simulink model "TTS2_EXT"  (R2025b)
settings: Solver=FixedStepAuto  StartTime=0.0  StopTime=inf  FixedStep=0.01  RelTol=1e-3
model workspace (MAT data in the model file):
  amp_f1 = -100
  amp_f10 = 0.5
  amp_f11 = -0.1
  amp_f12 = 1
  amp_f13 = 0.5
  amp_f14 = -20
  amp_f15 = 0.5
  amp_f16 = 0.5
  amp_f17 = 20
  amp_f18 = -30
  amp_f19 = 0.1
  amp_f2 = -20
  amp_f20 = -20
  amp_f21 = 20
  amp_f3 = -30
  amp_f4 = -30
  amp_f5 = -10
  amp_f51 = -10
  amp_f52 = -30
  amp_f53 = -30
  amp_f54 = 20
  amp_f55 = -100
  amp_f6 = -30
  amp_f7 = -30
  amp_f8 = -30
  amp_f9 = 1
  from_f1 = 570
  from_f10 = 5970
  from_f11 = 6570
  from_f12 = 7170
  from_f13 = 7770
  from_f14 = 8370
  from_f15 = 8970
  from_f16 = 9570
  from_f17 = 10170
  from_f18 = 10770
  from_f19 = 11370
  from_f2 = 1170
  from_f20 = 11970
  from_f21 = 12570
  from_f3 = 1770
  from_f4 = 2370
  from_f5 = 2970
  from_f51 = 13170
  from_f52 = 13770
  from_f53 = 14370
  from_f54 = 14970
  from_f55 = 15570
  from_f6 = 3570
  from_f7 = 4170
  from_f8 = 4770
  from_f9 = 5370
libraries: lab310_library x26, neural x15, simulink x4, opclib x3, fuzblock x1
(part 3 of 3)

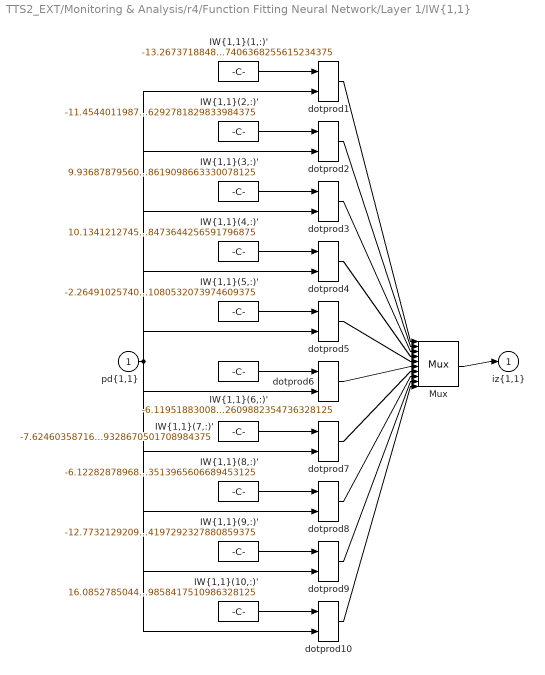
== system TTS2_EXT/Monitoring & Analysis/r4/Function Fitting Neural Network/Layer 1/IW{1,1} ==
  "pd{1,1}" : Inport  PortDimensions=1
      mask Display: e = 0.06;c1 = [120 230 180]/255;c2 = ([120 230 180]+0)/(256+128);c3 = ([120 230 180]+128)/(256+128);patch([0 1 1 0],[0 0 1 1],c1);patch([0 1 1 1-e 1-e 0+e],[0 0 1 1-e 0+e 0+e],c2);patch([0 0 1 1-e 0+e 0+e],[0 1 1 1-e 1-e 0+e],c3);plot([0 1 1 0 0],[0 0 1 1 0]);
  "IW{1,1}(1,:)'" : Constant  Value=-13.267371884858700781251172884367406368255615234375
      mask Display: e = 0.06;c1 = [120 150 230]/255;c2 = ([120 150 230]+0)/383;c3 = ([120 150 230]+128)/383;patch([0 1 1 0],[0 0 1 1],c1);patch([0 1 1 1-e 1-e 0+e],[0 0 1 1-e 0+e 0+e],c2);patch([0 0 1 1-e 0+e 0+e],[0 1 1 1-e 1-e 0+e],c3);plot([0 1 1 0 0],[0 0 1 1 0]);disp('Weights');
  "IW{1,1}(10,:)'" : Constant  Value=16.085278504446240077641050447709858417510986328125
      mask Display: e = 0.06;c1 = [120 150 230]/255;c2 = ([120 150 230]+0)/383;c3 = ([120 150 230]+128)/383;patch([0 1 1 0],[0 0 1 1],c1);patch([0 1 1 1-e 1-e 0+e],[0 0 1 1-e 0+e 0+e],c2);patch([0 0 1 1-e 0+e 0+e],[0 1 1 1-e 1-e 0+e],c3);plot([0 1 1 0 0],[0 0 1 1 0]);disp('Weights');
  "IW{1,1}(2,:)'" : Constant  Value=-11.4544011987529952278919154196046292781829833984375
      mask Display: e = 0.06;c1 = [120 150 230]/255;c2 = ([120 150 230]+0)/383;c3 = ([120 150 230]+128)/383;patch([0 1 1 0],[0 0 1 1],c1);patch([0 1 1 1-e 1-e 0+e],[0 0 1 1-e 0+e 0+e],c2);patch([0 0 1 1-e 0+e 0+e],[0 1 1 1-e 1-e 0+e],c3);plot([0 1 1 0 0],[0 0 1 1 0]);disp('Weights');
  "IW{1,1}(3,:)'" : Constant  Value=9.936878795604048519862772081978619098663330078125
      mask Display: e = 0.06;c1 = [120 150 230]/255;c2 = ([120 150 230]+0)/383;c3 = ([120 150 230]+128)/383;patch([0 1 1 0],[0 0 1 1],c1);patch([0 1 1 1-e 1-e 0+e],[0 0 1 1-e 0+e 0+e],c2);patch([0 0 1 1-e 0+e 0+e],[0 1 1 1-e 1-e 0+e],c3);plot([0 1 1 0 0],[0 0 1 1 0]);disp('Weights');
  "IW{1,1}(4,:)'" : Constant  Value=10.1341212745394653182984257000498473644256591796875
      mask Display: e = 0.06;c1 = [120 150 230]/255;c2 = ([120 150 230]+0)/383;c3 = ([120 150 230]+128)/383;patch([0 1 1 0],[0 0 1 1],c1);patch([0 1 1 1-e 1-e 0+e],[0 0 1 1-e 0+e 0+e],c2);patch([0 0 1 1-e 0+e 0+e],[0 1 1 1-e 1-e 0+e],c3);plot([0 1 1 0 0],[0 0 1 1 0]);disp('Weights');
  "IW{1,1}(5,:)'" : Constant  Value=-2.26491025740641926944363149232231080532073974609375
      mask Display: e = 0.06;c1 = [120 150 230]/255;c2 = ([120 150 230]+0)/383;c3 = ([120 150 230]+128)/383;patch([0 1 1 0],[0 0 1 1],c1);patch([0 1 1 1-e 1-e 0+e],[0 0 1 1-e 0+e 0+e],c2);patch([0 0 1 1-e 0+e 0+e],[0 1 1 1-e 1-e 0+e],c3);plot([0 1 1 0 0],[0 0 1 1 0]);disp('Weights');
  "IW{1,1}(6,:)'" : Constant  Value=-6.1195188300888077037598122842609882354736328125
      mask Display: e = 0.06;c1 = [120 150 230]/255;c2 = ([120 150 230]+0)/383;c3 = ([120 150 230]+128)/383;patch([0 1 1 0],[0 0 1 1],c1);patch([0 1 1 1-e 1-e 0+e],[0 0 1 1-e 0+e 0+e],c2);patch([0 0 1 1-e 0+e 0+e],[0 1 1 1-e 1-e 0+e],c3);plot([0 1 1 0 0],[0 0 1 1 0]);disp('Weights');
  "IW{1,1}(7,:)'" : Constant  Value=-7.62460358716090436104195759980939328670501708984375
      mask Display: e = 0.06;c1 = [120 150 230]/255;c2 = ([120 150 230]+0)/383;c3 = ([120 150 230]+128)/383;patch([0 1 1 0],[0 0 1 1],c1);patch([0 1 1 1-e 1-e 0+e],[0 0 1 1-e 0+e 0+e],c2);patch([0 0 1 1-e 0+e 0+e],[0 1 1 1-e 1-e 0+e],c3);plot([0 1 1 0 0],[0 0 1 1 0]);disp('Weights');
  "IW{1,1}(8,:)'" : Constant  Value=-6.122828789688373518629305181093513965606689453125
      mask Display: e = 0.06;c1 = [120 150 230]/255;c2 = ([120 150 230]+0)/383;c3 = ([120 150 230]+128)/383;patch([0 1 1 0],[0 0 1 1],c1);patch([0 1 1 1-e 1-e 0+e],[0 0 1 1-e 0+e 0+e],c2);patch([0 0 1 1-e 0+e 0+e],[0 1 1 1-e 1-e 0+e],c3);plot([0 1 1 0 0],[0 0 1 1 0]);disp('Weights');
  "IW{1,1}(9,:)'" : Constant  Value=-12.7732129209851503759409752092324197292327880859375
      mask Display: e = 0.06;c1 = [120 150 230]/255;c2 = ([120 150 230]+0)/383;c3 = ([120 150 230]+128)/383;patch([0 1 1 0],[0 0 1 1],c1);patch([0 1 1 1-e 1-e 0+e],[0 0 1 1-e 0+e 0+e],c2);patch([0 0 1 1-e 0+e 0+e],[0 1 1 1-e 1-e 0+e],c3);plot([0 1 1 0 0],[0 0 1 1 0]);disp('Weights');
  Mux : Mux  Inputs=10
      mask Display: e = 0.06;c1 = [120 150 230]/255;c2 = ([120 150 230]+0)/383;c3 = ([120 150 230]+128)/383;patch([0 1 1 0],[0 0 1 1],c1);patch([0 1 1 1-e 1-e 0+e],[0 0 1 1-e 0+e 0+e],c2);patch([0 0 1 1-e 0+e 0+e],[0 1 1 1-e 1-e 0+e],c3);plot([0 1 1 0 0],[0 0 1 1 0]);disp('Mux');
  dotprod{1..10} (10 alike) : neural/Weight Functions/dotprod
  "iz{1,1}" : Outport
      mask Display: e = 0.06;c1 = [120 230 180]/255;c2 = ([120 230 180]+0)/(256+128);c3 = ([120 230 180]+128)/(256+128);patch([0 1 1 0],[0 0 1 1],c1);patch([0 1 1 1-e 1-e 0+e],[0 0 1 1-e 0+e 0+e],c2);patch([0 0 1 1-e 0+e 0+e],[0 1 1 1-e 1-e 0+e],c3);plot([0 1 1 0 0],[0 0 1 1 0]);
  wires:
  "IW{1,1}(1,:)'"/1 -> dotprod1/1
  "pd{1,1}"/1 -> dotprod1/2, dotprod2/2, dotprod3/2, dotprod4/2, dotprod5/2, dotprod6/2, dotprod7/2, dotprod8/2, dotprod9/2, dotprod10/2
  dotprod1/1 -> Mux/1
  "IW{1,1}(2,:)'"/1 -> dotprod2/1
  dotprod2/1 -> Mux/2
  "IW{1,1}(3,:)'"/1 -> dotprod3/1
  dotprod3/1 -> Mux/3
  "IW{1,1}(4,:)'"/1 -> dotprod4/1
  dotprod4/1 -> Mux/4
  "IW{1,1}(5,:)'"/1 -> dotprod5/1
  dotprod5/1 -> Mux/5
  "IW{1,1}(6,:)'"/1 -> dotprod6/1
  dotprod6/1 -> Mux/6
  "IW{1,1}(7,:)'"/1 -> dotprod7/1
  dotprod7/1 -> Mux/7
  "IW{1,1}(8,:)'"/1 -> dotprod8/1
  dotprod8/1 -> Mux/8
  "IW{1,1}(9,:)'"/1 -> dotprod9/1
  dotprod9/1 -> Mux/9
  "IW{1,1}(10,:)'"/1 -> dotprod10/1
  dotprod10/1 -> Mux/10
  Mux/1 -> "iz{1,1}"/1

== system TTS2_EXT/Monitoring & Analysis/r4/Function Fitting Neural Network/Layer 2/Delays 1 ==
  "p{2}" : Inport  PortDimensions=10
      mask Display: e = 0.06;c1 = [120 230 180]/255;c2 = ([120 230 180]+0)/(256+128);c3 = ([120 230 180]+128)/(256+128);patch([0 1 1 0],[0 0 1 1],c1);patch([0 1 1 1-e 1-e 0+e],[0 0 1 1-e 0+e 0+e],c2);patch([0 0 1 1-e 0+e 0+e],[0 1 1 1-e 1-e 0+e],c3);plot([0 1 1 0 0],[0 0 1 1 0]);
  mux : Mux  Inputs=1
      mask Display: e = 0.06;c1 = [120 150 230]/255;c2 = ([120 150 230]+0)/383;c3 = ([120 150 230]+128)/383;patch([0 1 1 0],[0 0 1 1],c1);patch([0 1 1 1-e 1-e 0+e],[0 0 1 1-e 0+e 0+e],c2);patch([0 0 1 1-e 0+e 0+e],[0 1 1 1-e 1-e 0+e],c3);plot([0 1 1 0 0],[0 0 1 1 0]);disp('Mux')
  "pd{2,1}" : Outport
      mask Display: e = 0.06;c1 = [120 230 180]/255;c2 = ([120 230 180]+0)/(256+128);c3 = ([120 230 180]+128)/(256+128);patch([0 1 1 0],[0 0 1 1],c1);patch([0 1 1 1-e 1-e 0+e],[0 0 1 1-e 0+e 0+e],c2);patch([0 0 1 1-e 0+e 0+e],[0 1 1 1-e 1-e 0+e],c3);plot([0 1 1 0 0],[0 0 1 1 0]);
  wires:
  "p{2}"/1 -> mux/1
  mux/1 -> "pd{2,1}"/1

== system TTS2_EXT/Monitoring & Analysis/r4/Function Fitting Neural Network/Layer 2/LW{2,1} ==
  "ad{2,1}" : Inport  PortDimensions=10
      mask Display: e = 0.06;c1 = [120 230 180]/255;c2 = ([120 230 180]+0)/(256+128);c3 = ([120 230 180]+128)/(256+128);patch([0 1 1 0],[0 0 1 1],c1);patch([0 1 1 1-e 1-e 0+e],[0 0 1 1-e 0+e 0+e],c2);patch([0 0 1 1-e 0+e 0+e],[0 1 1 1-e 1-e 0+e],c3);plot([0 1 1 0 0],[0 0 1 1 0]);
  "IW{2,1}(1,:)'" : Constant  Value=[-0.0273434432413987814347589022645479417406022548675537109375;-0.04215844327802921454040330218049348331987857818603515625;0.0296321635772760529070612989244182244874536991119384765625;0.019112043841627852913678253798934747464954853057861328125;-0.282504725481045382284861489097238518297672271728515625;-0.0481063819827808047957518056136905215680599212646484375;-0.06977041381876440684361995181461679749190807342529296875;-0.179432033501076226844617167444084770977497100830078125;-0.10706544318229176127044155464318464510142803192138671875;1.657272038694669991087948801578022539615631103515625]
      mask Display: e = 0.06;c1 = [120 150 230]/255;c2 = ([120 150 230]+0)/383;c3 = ([120 150 230]+128)/383;patch([0 1 1 0],[0 0 1 1],c1);patch([0 1 1 1-e 1-e 0+e],[0 0 1 1-e 0+e 0+e],c2);patch([0 0 1 1-e 0+e 0+e],[0 1 1 1-e 1-e 0+e],c3);plot([0 1 1 0 0],[0 0 1 1 0]);disp('weights');
  Mux : Mux  Inputs=1
      mask Display: e = 0.06;c1 = [120 150 230]/255;c2 = ([120 150 230]+0)/383;c3 = ([120 150 230]+128)/383;patch([0 1 1 0],[0 0 1 1],c1);patch([0 1 1 1-e 1-e 0+e],[0 0 1 1-e 0+e 0+e],c2);patch([0 0 1 1-e 0+e 0+e],[0 1 1 1-e 1-e 0+e],c3);plot([0 1 1 0 0],[0 0 1 1 0]);disp('Mux');
  dotprod1 : neural/Weight Functions/dotprod
  "lz{2,1}" : Outport
      mask Display: e = 0.06;c1 = [120 230 180]/255;c2 = ([120 230 180]+0)/(256+128);c3 = ([120 230 180]+128)/(256+128);patch([0 1 1 0],[0 0 1 1],c1);patch([0 1 1 1-e 1-e 0+e],[0 0 1 1-e 0+e 0+e],c2);patch([0 0 1 1-e 0+e 0+e],[0 1 1 1-e 1-e 0+e],c3);plot([0 1 1 0 0],[0 0 1 1 0]);
  wires:
  "IW{2,1}(1,:)'"/1 -> dotprod1/1
  "ad{2,1}"/1 -> dotprod1/2
  dotprod1/1 -> Mux/1
  Mux/1 -> "lz{2,1}"/1

== system TTS2_EXT/TTS2/Disturbance: Pump+pipe+control valve/VB/Valve/liniowa ==
  CV : Inport
  dP : Inport  Port=2
  param : Inport  Port=3
  Bus Selector : BusSelector  OutputSignals=signal4,signal2,signal1,signal3
  Fcn : Fcn  Expr=u(2)*(u(1)-1)
  Fcn1 : Fcn  Expr=sqrt(u(1)/u(2))/10
  Math Function : Math  SignedPower=on
  Mux : Mux  Inputs=2
  Mux1 : Mux  Inputs=2
  Product : Product  Inputs=*/***
  F : Outport  VectorParamsAs1DForOutWhenUnconnected=off
  wires:
  param/1 -> Bus Selector/1
  Fcn/1 -> Math Function/1
  Math Function/1 -> Product/1
  Product/1 -> F/1
  Mux/1 -> Fcn/1
  Mux1/1 -> Fcn1/1
  dP/1 -> Mux1/1
  Bus Selector/2 -> Mux/2  "<signal2>"
  Bus Selector/3 -> Product/3  "<signal1>"
  Fcn1/1 -> Product/5
  Bus Selector/4 -> Mux1/2  "<signal3>"
  Bus Selector/1 -> Product/2, Mux/1  "<signal4>"
  CV/1 -> Product/4

== system TTS2_EXT/TTS2/Disturbance: Pump+pipe+control valve/VB/Valve/stałoproc. ==
  CV : Inport
  dP : Inport  Port=2
  param : Inport  Port=3
  Bus Selector : BusSelector  OutputSignals=signal2,signal1,signal3
  Fcn : Fcn  Expr=u(2)*(u(1)-1)
  Fcn1 : Fcn  Expr=sqrt(u(1)/u(2))/10
  Math Function : Math  SignedPower=on
  Mux : Mux  Inputs=2
  Mux1 : Mux  Inputs=2
  Product : Product  Inputs=3
  F : Outport  VectorParamsAs1DForOutWhenUnconnected=off
  wires:
  param/1 -> Bus Selector/1
  Fcn/1 -> Math Function/1
  Math Function/1 -> Product/1
  Product/1 -> F/1
  CV/1 -> Mux/1
  Mux/1 -> Fcn/1
  Mux1/1 -> Fcn1/1
  dP/1 -> Mux1/1
  Bus Selector/1 -> Mux/2  "<signal2>"
  Bus Selector/2 -> Product/2  "<signal1>"
  Fcn1/1 -> Product/3
  Bus Selector/3 -> Mux1/2  "<signal3>"

== system TTS2_EXT/TTS2/Pump+pipe+control valve/V1/Valve/liniowa ==
  CV : Inport
  dP : Inport  Port=2
  param : Inport  Port=3
  Bus Selector : BusSelector  OutputSignals=signal4,signal2,signal1,signal3
  Fcn : Fcn  Expr=u(2)*(u(1)-1)
  Fcn1 : Fcn  Expr=sqrt(u(1)/u(2))/10
  Math Function : Math  SignedPower=on
  Mux : Mux  Inputs=2
  Mux1 : Mux  Inputs=2
  Product : Product  Inputs=*/***
  F : Outport  VectorParamsAs1DForOutWhenUnconnected=off
  wires:
  param/1 -> Bus Selector/1
  Fcn/1 -> Math Function/1
  Math Function/1 -> Product/1
  Product/1 -> F/1
  Mux/1 -> Fcn/1
  Mux1/1 -> Fcn1/1
  dP/1 -> Mux1/1
  Bus Selector/2 -> Mux/2  "<signal2>"
  Bus Selector/3 -> Product/3  "<signal1>"
  Fcn1/1 -> Product/5
  Bus Selector/4 -> Mux1/2  "<signal3>"
  Bus Selector/1 -> Product/2, Mux/1  "<signal4>"
  CV/1 -> Product/4

== system TTS2_EXT/TTS2/Pump+pipe+control valve/V1/Valve/stałoproc. ==
  CV : Inport
  dP : Inport  Port=2
  param : Inport  Port=3
  Bus Selector : BusSelector  OutputSignals=signal2,signal1,signal3
  Fcn : Fcn  Expr=u(2)*(u(1)-1)
  Fcn1 : Fcn  Expr=sqrt(u(1)/u(2))/10
  Math Function : Math  SignedPower=on
  Mux : Mux  Inputs=2
  Mux1 : Mux  Inputs=2
  Product : Product  Inputs=3
  F : Outport  VectorParamsAs1DForOutWhenUnconnected=off
  wires:
  param/1 -> Bus Selector/1
  Fcn/1 -> Math Function/1
  Math Function/1 -> Product/1
  Product/1 -> F/1
  CV/1 -> Mux/1
  Mux/1 -> Fcn/1
  Mux1/1 -> Fcn1/1
  dP/1 -> Mux1/1
  Bus Selector/1 -> Mux/2  "<signal2>"
  Bus Selector/2 -> Product/2  "<signal1>"
  Fcn1/1 -> Product/3
  Bus Selector/3 -> Mux1/2  "<signal3>"

== system TTS2_EXT/TTS2/Pump+pipe+control valve/V2/Valve/liniowa ==
  CV : Inport
  dP : Inport  Port=2
  param : Inport  Port=3
  Bus Selector : BusSelector  OutputSignals=signal4,signal2,signal1,signal3
  Fcn : Fcn  Expr=u(2)*(u(1)-1)
  Fcn1 : Fcn  Expr=sqrt(u(1)/u(2))/10
  Math Function : Math  SignedPower=on
  Mux : Mux  Inputs=2
  Mux1 : Mux  Inputs=2
  Product : Product  Inputs=*/***
  F : Outport  VectorParamsAs1DForOutWhenUnconnected=off
  wires:
  param/1 -> Bus Selector/1
  Fcn/1 -> Math Function/1
  Math Function/1 -> Product/1
  Product/1 -> F/1
  Mux/1 -> Fcn/1
  Mux1/1 -> Fcn1/1
  dP/1 -> Mux1/1
  Bus Selector/2 -> Mux/2  "<signal2>"
  Bus Selector/3 -> Product/3  "<signal1>"
  Fcn1/1 -> Product/5
  Bus Selector/4 -> Mux1/2  "<signal3>"
  Bus Selector/1 -> Product/2, Mux/1  "<signal4>"
  CV/1 -> Product/4

== system TTS2_EXT/TTS2/Pump+pipe+control valve/V2/Valve/stałoproc. ==
  CV : Inport
  dP : Inport  Port=2
  param : Inport  Port=3
  Bus Selector : BusSelector  OutputSignals=signal2,signal1,signal3
  Fcn : Fcn  Expr=u(2)*(u(1)-1)
  Fcn1 : Fcn  Expr=sqrt(u(1)/u(2))/10
  Math Function : Math  SignedPower=on
  Mux : Mux  Inputs=2
  Mux1 : Mux  Inputs=2
  Product : Product  Inputs=3
  F : Outport  VectorParamsAs1DForOutWhenUnconnected=off
  wires:
  param/1 -> Bus Selector/1
  Fcn/1 -> Math Function/1
  Math Function/1 -> Product/1
  Product/1 -> F/1
  CV/1 -> Mux/1
  Mux/1 -> Fcn/1
  Mux1/1 -> Fcn1/1
  dP/1 -> Mux1/1
  Bus Selector/1 -> Mux/2  "<signal2>"
  Bus Selector/2 -> Product/2  "<signal1>"
  Fcn1/1 -> Product/3
  Bus Selector/3 -> Mux1/2  "<signal3>"
